simulink model "simulinkPark"  (R2024a)
settings: Solver=VariableStepAuto  StartTime=0.0  StopTime=11.5667  RelTol=1e-3
values from neighbouring files (symbols this model uses):
  posX = [sampleTimes',position(:,1)]    [main.m]
  posY = [sampleTimes',position(:,2)]    [main.m]
  posYaw = [sampleTimes',yaw]    [main.m]
libraries: sim3dautolib x11, visionsinks x2, sim3dcameralib x1, sim3dlib x1
settings Model: Creator=6000022946  LastModifiedBy=Administrator
settings RTWCC: GPUComputeCapability=3.5

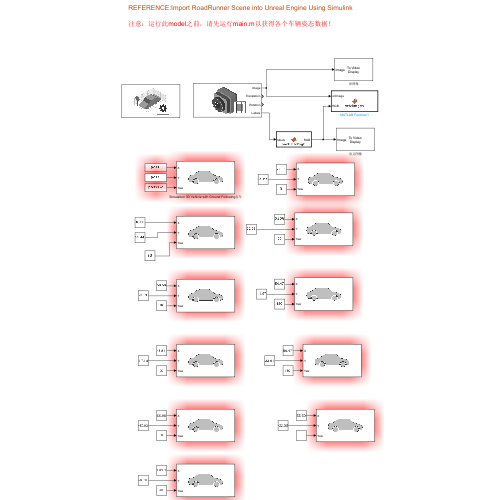
[thumbnail: Simulink's stored preview of the top-level diagram]
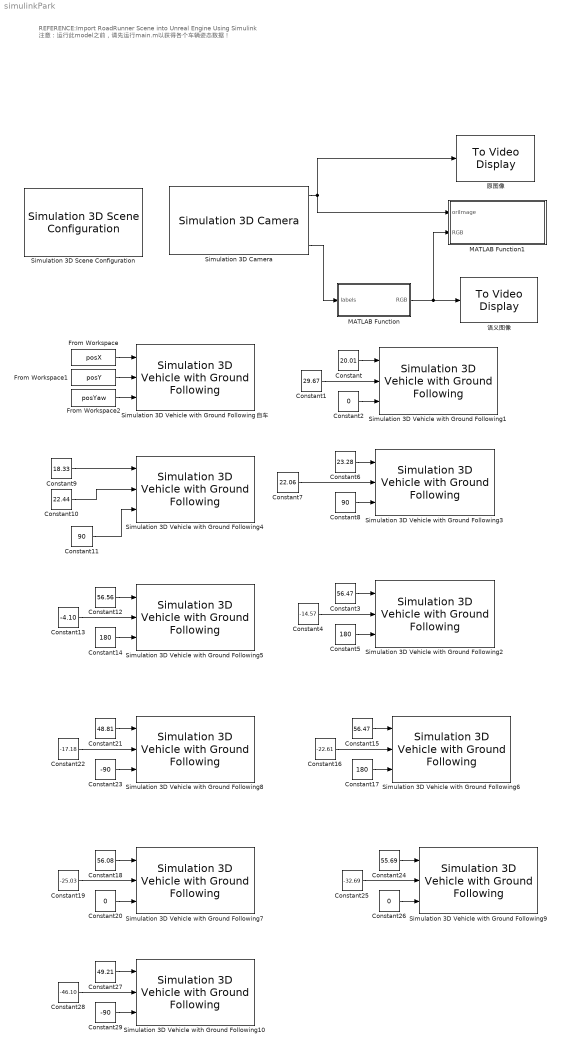
== system simulinkPark ==
  note: REFERENCE:Import RoadRunner Scene into Unreal Engine Using Simulink
      |
      | 注意：运行此model之前，请先运行main.m以获得各个车辆姿态数据！
  Constant : Constant  Value=20.01
  Constant1 : Constant  Value=29.67
  Constant10 : Constant  Value=22.44
  Constant11 : Constant  Value=90
  Constant12 : Constant  Value=56.56
  Constant13 : Constant  Value=-4.10
  Constant14 : Constant  Value=180
  Constant15 : Constant  Value=56.47
  Constant16 : Constant  Value=-22.61
  Constant17 : Constant  Value=180
  Constant18 : Constant  Value=56.08
  Constant19 : Constant  Value=-25.03
  Constant2 : Constant  Value=0
  Constant20 : Constant  Value=0
  Constant21 : Constant  Value=48.81
  Constant22 : Constant  Value=-17.18
  Constant23 : Constant  Value=-90
  Constant24 : Constant  Value=55.69
  Constant25 : Constant  Value=-32.69
  Constant26 : Constant  Value=0
  Constant27 : Constant  Value=49.21
  Constant28 : Constant  Value=-46.10
  Constant29 : Constant  Value=-90
  Constant3 : Constant  Value=56.47
  Constant4 : Constant  Value=-14.57
  Constant5 : Constant  Value=180
  Constant6 : Constant  Value=23.28
  Constant7 : Constant  Value=22.06
  Constant8 : Constant  Value=90
  Constant9 : Constant  Value=18.33
  From Workspace : FromWorkspace  VariableName=posX
  From Workspace1 : FromWorkspace  VariableName=posY
  From Workspace2 : FromWorkspace  VariableName=posYaw
  MATLAB Function : MATLAB Function  TreatAsAtomicUnit=on
  MATLAB Function1 : MATLAB Function  TreatAsAtomicUnit=on
  Simulation 3D Camera : sim3dcameralib/Simulation 3D Camera  Priority=1  sensorTag=Sim3dSensor5  sensorId=5  sensorName=Sim3dSensor5  vehTagList={'Scene Origin';'SimulinkVehicle10';'SimulinkVehicle11';'SimulinkVehicle12';'SimulinkVehicle13';'SimulinkVehicle4';'SimulinkVehicle5';'SimulinkVehicle6';'SimulinkVehicle7';'SimulinkVehicle8';'SimulinkVehicle9';'myEgoVehicle'}  vehTag=myEgoVehicle  mountLoc=Origin  offsetFlag=on  tmountOffset=[0, 0, 20]  extTmount=off  rmountOffset=[0, 90, 0]  extRmount=off  FocalLength=[1109, 1109]  OpticalCenter=[640, 360]  ImageSize=[720, 1280]  RadialDistortion=[0, 0]  TangentialDistortion=[0, 0]  SensorSkew=0  DepthOutportEnabled=off  SemanticOutportEnabled=on  TransformOutportEnabled=on  SampleTime=-1  mountPoint=[0 0 20]  mountOrientation=[0 -90 0]  aMode=3  ID=5
      settings: LibrarySourceBlock=drivingsim3d/Simulation 3D Camera
  Simulation 3D Scene Configuration : sim3dlib/Simulation 3D Scene Configuration  Priority=0  ProjectFormat=RoadRunner  SceneDesc=Straight road  ProjectName=C:\Program Files\MATLAB\R2024a\toolbox\shared\sim3d_projects\automotive_project_windows\UE\WindowsNoEditor\VehicleSimulation.exe  ScenePath=/Game/Maps/HwStrght  RoadRunnerProjectPath=./Exports/mySampleParking.fbx  EnableOpenDRIVE=off  vehTagList={'Custom';'Scene Origin';'SimulinkVehicle10';'SimulinkVehicle11';'SimulinkVehicle12';'SimulinkVehicle13';'SimulinkVehicle4';'SimulinkVehicle5';'SimulinkVehicle6';'SimulinkVehicle7';'SimulinkVehicle8';'SimulinkVehicle9';'myEgoVehicle'}  vehTag=Custom  FreeCameraInitialTranslation=[50, 0, 200]  FreeCameraDefaultInitialTranslation=[-6, 0, 2]  FreeCameraInitialRotation=[0, -90, 0]  FreeCameraDefaultInitialRotation=[0, -15, 0]  OpVisEn=off  Ts=1/60  EnableWindow=on  EnableRemoteAccess=off  EnableWeather=on  SunAzimuth=90  SunAltitude=40.0  EnableGeospatialSun=off  Latitude=0  Longitude=0  Date=2023-01-01  Time=10:30:00  GeoTimeZone=-5.0  SunDaylightSaving=off  wind=1  clouds=10  EnableVolumetricClouds=off  CloudCoverage=0  CloudAltitude=6  fog=57.0  rain=0.0  RaindropsEffect=off  SnowDensity=0  EnableGeospatial=off  UseTrueOrigin=off  OriginHeight=200  OriginLatitude=40.744652  OriginLongitude=-73.988864  MapStyle=Aerial  AdditionalAssetIDs=[]  UseAdvancedSunSky=off  SolarTime=11  TimeZone=-5  Day=21  Month=9  Year=2022  UseDaylightSavingTime=on  DSTStartDay=10  DSTStartMonth=3  DSTEndDay=3  DSTEndMonth=11  DSTSwitchHour=2  sensorTag=MainCamera1  sensorId=1  sensorName=MainCamera1  mountLoc=Origin  offsetFlag=off  tmountOffset=[0, 0, 0]  rmountOffset=[0, 0, 0]  HorizontalResolution=1280  VerticalResolution=720  HorizontalFOV=60  mountPoint=[0 0 0]  mountOrientation=[0 0 0]  aMode=3  ID=1  GeoTrigger=Inactive
      settings: LibrarySourceBlock=drivingsim3d/Simulation 3D Scene Configuration
  Simulation 3D Vehicle with Ground Following1 : sim3dautolib/Simulation 3D Vehicle with Ground Following  Priority=-1  PassVehMesh=Sport utility vehicle  MeshPath=/MathWorksAutomotiveContent/Vehicles/Muscle/Meshes/SK_MuscleCar.SK_MuscleCar  TrackWidth=1.9  WheelBase=3  WheelRadius=0.35  VehColor=Orange  InitialPos=[posX(1,2), posY(1,2), 0]  InitialRot=[0, 0, posYaw(1,2)]  ActorName=SimulinkVehicle4  SampleTime=-1  ActorType=SimulinkVehicle  ID=4  aMode=3  ActorTag=SimulinkVehicle4  CoordinateScheme=ISO  VehLightsControl=off  HeadlightColor=[ 1, 1, 1 ]  HighBeamIntensity=100000  LowBeamIntensity=60000  HighBeamConeAngle=70  LowBeamConeAngle=70  LeftHeadlightOrientation=[ 0, 0 ]  RightHeadlightOrientation=[ 0, 0 ]  BrakelightIntensity=500  ReverselightIntensity=500  SignallightIntensity=500  SignallightPeriod=1  SignalPulseWidth=50  TransformOutportEnabled=off
      settings: LibrarySourceBlock=drivingsim3d/Simulation 3D Vehicle with Ground Following
  Simulation 3D Vehicle with Ground Following10 : sim3dautolib/Simulation 3D Vehicle with Ground Following  Priority=-1  PassVehMesh=Muscle car  MeshPath=/MathWorksAutomotiveContent/Vehicles/Muscle/Meshes/SK_MuscleCar.SK_MuscleCar  TrackWidth=1.9  WheelBase=3  WheelRadius=0.35  VehColor=White  InitialPos=[posX(1,2), posY(1,2), 0]  InitialRot=[0, 0, posYaw(1,2)]  ActorName=SimulinkVehicle13  SampleTime=-1  ActorType=SimulinkVehicle  ID=13  aMode=3  ActorTag=SimulinkVehicle13  CoordinateScheme=ISO  VehLightsControl=off  HeadlightColor=[ 1, 1, 1 ]  HighBeamIntensity=100000  LowBeamIntensity=60000  HighBeamConeAngle=70  LowBeamConeAngle=70  LeftHeadlightOrientation=[ 0, 0 ]  RightHeadlightOrientation=[ 0, 0 ]  BrakelightIntensity=500  ReverselightIntensity=500  SignallightIntensity=500  SignallightPeriod=1  SignalPulseWidth=50  TransformOutportEnabled=off
      settings: LibrarySourceBlock=drivingsim3d/Simulation 3D Vehicle with Ground Following
  Simulation 3D Vehicle with Ground Following2 : sim3dautolib/Simulation 3D Vehicle with Ground Following  Priority=-1  PassVehMesh=Hatchback  MeshPath=/MathWorksAutomotiveContent/Vehicles/Muscle/Meshes/SK_MuscleCar.SK_MuscleCar  TrackWidth=1.9  WheelBase=3  WheelRadius=0.35  VehColor=Yellow  InitialPos=[posX(1,2), posY(1,2), 0]  InitialRot=[0, 0, posYaw(1,2)]  ActorName=SimulinkVehicle5  SampleTime=-1  ActorType=SimulinkVehicle  ID=5  aMode=3  ActorTag=SimulinkVehicle5  CoordinateScheme=ISO  VehLightsControl=off  HeadlightColor=[ 1, 1, 1 ]  HighBeamIntensity=100000  LowBeamIntensity=60000  HighBeamConeAngle=70  LowBeamConeAngle=70  LeftHeadlightOrientation=[ 0, 0 ]  RightHeadlightOrientation=[ 0, 0 ]  BrakelightIntensity=500  ReverselightIntensity=500  SignallightIntensity=500  SignallightPeriod=1  SignalPulseWidth=50  TransformOutportEnabled=off
      settings: LibrarySourceBlock=drivingsim3d/Simulation 3D Vehicle with Ground Following
  Simulation 3D Vehicle with Ground Following3 : sim3dautolib/Simulation 3D Vehicle with Ground Following  Priority=-1  PassVehMesh=Sedan  MeshPath=/MathWorksAutomotiveContent/Vehicles/Muscle/Meshes/SK_MuscleCar.SK_MuscleCar  TrackWidth=1.9  WheelBase=3  WheelRadius=0.35  VehColor=White  InitialPos=[posX(1,2), posY(1,2), 0]  InitialRot=[0, 0, posYaw(1,2)]  ActorName=SimulinkVehicle6  SampleTime=-1  ActorType=SimulinkVehicle  ID=6  aMode=3  ActorTag=SimulinkVehicle6  CoordinateScheme=ISO  VehLightsControl=off  HeadlightColor=[ 1, 1, 1 ]  HighBeamIntensity=100000  LowBeamIntensity=60000  HighBeamConeAngle=70  LowBeamConeAngle=70  LeftHeadlightOrientation=[ 0, 0 ]  RightHeadlightOrientation=[ 0, 0 ]  BrakelightIntensity=500  ReverselightIntensity=500  SignallightIntensity=500  SignallightPeriod=1  SignalPulseWidth=50  TransformOutportEnabled=off
      settings: LibrarySourceBlock=drivingsim3d/Simulation 3D Vehicle with Ground Following
  Simulation 3D Vehicle with Ground Following4 : sim3dautolib/Simulation 3D Vehicle with Ground Following  Priority=-1  PassVehMesh=Sedan  MeshPath=/MathWorksAutomotiveContent/Vehicles/Muscle/Meshes/SK_MuscleCar.SK_MuscleCar  TrackWidth=1.9  WheelBase=3  WheelRadius=0.35  VehColor=Blue  InitialPos=[posX(1,2), posY(1,2), 0]  InitialRot=[0, 0, posYaw(1,2)]  ActorName=SimulinkVehicle7  SampleTime=-1  ActorType=SimulinkVehicle  ID=7  aMode=3  ActorTag=SimulinkVehicle7  CoordinateScheme=ISO  VehLightsControl=off  HeadlightColor=[ 1, 1, 1 ]  HighBeamIntensity=100000  LowBeamIntensity=60000  HighBeamConeAngle=70  LowBeamConeAngle=70  LeftHeadlightOrientation=[ 0, 0 ]  RightHeadlightOrientation=[ 0, 0 ]  BrakelightIntensity=500  ReverselightIntensity=500  SignallightIntensity=500  SignallightPeriod=1  SignalPulseWidth=50  TransformOutportEnabled=off
      settings: LibrarySourceBlock=drivingsim3d/Simulation 3D Vehicle with Ground Following
  Simulation 3D Vehicle with Ground Following5 : sim3dautolib/Simulation 3D Vehicle with Ground Following  Priority=-1  PassVehMesh=Sedan  MeshPath=/MathWorksAutomotiveContent/Vehicles/Muscle/Meshes/SK_MuscleCar.SK_MuscleCar  TrackWidth=1.9  WheelBase=3  WheelRadius=0.35  VehColor=White  InitialPos=[posX(1,2), posY(1,2), 0]  InitialRot=[0, 0, posYaw(1,2)]  ActorName=SimulinkVehicle8  SampleTime=-1  ActorType=SimulinkVehicle  ID=8  aMode=3  ActorTag=SimulinkVehicle8  CoordinateScheme=ISO  VehLightsControl=off  HeadlightColor=[ 1, 1, 1 ]  HighBeamIntensity=100000  LowBeamIntensity=60000  HighBeamConeAngle=70  LowBeamConeAngle=70  LeftHeadlightOrientation=[ 0, 0 ]  RightHeadlightOrientation=[ 0, 0 ]  BrakelightIntensity=500  ReverselightIntensity=500  SignallightIntensity=500  SignallightPeriod=1  SignalPulseWidth=50  TransformOutportEnabled=off
      settings: LibrarySourceBlock=drivingsim3d/Simulation 3D Vehicle with Ground Following
  Simulation 3D Vehicle with Ground Following6 : sim3dautolib/Simulation 3D Vehicle with Ground Following  Priority=-1  PassVehMesh=Muscle car  MeshPath=/MathWorksAutomotiveContent/Vehicles/Muscle/Meshes/SK_MuscleCar.SK_MuscleCar  TrackWidth=1.9  WheelBase=3  WheelRadius=0.35  VehColor=White  InitialPos=[posX(1,2), posY(1,2), 0]  InitialRot=[0, 0, posYaw(1,2)]  ActorName=SimulinkVehicle9  SampleTime=-1  ActorType=SimulinkVehicle  ID=9  aMode=3  ActorTag=SimulinkVehicle9  CoordinateScheme=ISO  VehLightsControl=off  HeadlightColor=[ 1, 1, 1 ]  HighBeamIntensity=100000  LowBeamIntensity=60000  HighBeamConeAngle=70  LowBeamConeAngle=70  LeftHeadlightOrientation=[ 0, 0 ]  RightHeadlightOrientation=[ 0, 0 ]  BrakelightIntensity=500  ReverselightIntensity=500  SignallightIntensity=500  SignallightPeriod=1  SignalPulseWidth=50  TransformOutportEnabled=off
      settings: LibrarySourceBlock=drivingsim3d/Simulation 3D Vehicle with Ground Following
  Simulation 3D Vehicle with Ground Following7 : sim3dautolib/Simulation 3D Vehicle with Ground Following  Priority=-1  PassVehMesh=Small pickup truck  MeshPath=/MathWorksAutomotiveContent/Vehicles/Muscle/Meshes/SK_MuscleCar.SK_MuscleCar  TrackWidth=1.9  WheelBase=3  WheelRadius=0.35  VehColor=Black  InitialPos=[posX(1,2), posY(1,2), 0]  InitialRot=[0, 0, posYaw(1,2)]  ActorName=SimulinkVehicle10  SampleTime=-1  ActorType=SimulinkVehicle  ID=10  aMode=3  ActorTag=SimulinkVehicle10  CoordinateScheme=ISO  VehLightsControl=off  HeadlightColor=[ 1, 1, 1 ]  HighBeamIntensity=100000  LowBeamIntensity=60000  HighBeamConeAngle=70  LowBeamConeAngle=70  LeftHeadlightOrientation=[ 0, 0 ]  RightHeadlightOrientation=[ 0, 0 ]  BrakelightIntensity=500  ReverselightIntensity=500  SignallightIntensity=500  SignallightPeriod=1  SignalPulseWidth=50  TransformOutportEnabled=off
      settings: LibrarySourceBlock=drivingsim3d/Simulation 3D Vehicle with Ground Following
  Simulation 3D Vehicle with Ground Following8 : sim3dautolib/Simulation 3D Vehicle with Ground Following  Priority=-1  PassVehMesh=Box truck  MeshPath=/MathWorksAutomotiveContent/Vehicles/Muscle/Meshes/SK_MuscleCar.SK_MuscleCar  TrackWidth=1.9  WheelBase=3  WheelRadius=0.35  VehColor=Green  InitialPos=[posX(1,2), posY(1,2), 0]  InitialRot=[0, 0, posYaw(1,2)]  ActorName=SimulinkVehicle11  SampleTime=-1  ActorType=SimulinkVehicle  ID=11  aMode=3  ActorTag=SimulinkVehicle11  CoordinateScheme=ISO  VehLightsControl=off  HeadlightColor=[ 1, 1, 1 ]  HighBeamIntensity=100000  LowBeamIntensity=60000  HighBeamConeAngle=70  LowBeamConeAngle=70  LeftHeadlightOrientation=[ 0, 0 ]  RightHeadlightOrientation=[ 0, 0 ]  BrakelightIntensity=500  ReverselightIntensity=500  SignallightIntensity=500  SignallightPeriod=1  SignalPulseWidth=50  TransformOutportEnabled=off
      settings: LibrarySourceBlock=drivingsim3d/Simulation 3D Vehicle with Ground Following
  Simulation 3D Vehicle with Ground Following9 : sim3dautolib/Simulation 3D Vehicle with Ground Following  Priority=-1  PassVehMesh=Small pickup truck  MeshPath=/MathWorksAutomotiveContent/Vehicles/Muscle/Meshes/SK_MuscleCar.SK_MuscleCar  TrackWidth=1.9  WheelBase=3  WheelRadius=0.35  VehColor=White  InitialPos=[posX(1,2), posY(1,2), 0]  InitialRot=[0, 0, posYaw(1,2)]  ActorName=SimulinkVehicle12  SampleTime=-1  ActorType=SimulinkVehicle  ID=12  aMode=3  ActorTag=SimulinkVehicle12  CoordinateScheme=ISO  VehLightsControl=off  HeadlightColor=[ 1, 1, 1 ]  HighBeamIntensity=100000  LowBeamIntensity=60000  HighBeamConeAngle=70  LowBeamConeAngle=70  LeftHeadlightOrientation=[ 0, 0 ]  RightHeadlightOrientation=[ 0, 0 ]  BrakelightIntensity=500  ReverselightIntensity=500  SignallightIntensity=500  SignallightPeriod=1  SignalPulseWidth=50  TransformOutportEnabled=off
      settings: LibrarySourceBlock=drivingsim3d/Simulation 3D Vehicle with Ground Following
  Simulation 3D Vehicle with Ground Following自车 : sim3dautolib/Simulation 3D Vehicle with Ground Following  Priority=-1  PassVehMesh=Muscle car  MeshPath=/MathWorksAutomotiveContent/Vehicles/Muscle/Meshes/SK_MuscleCar.SK_MuscleCar  TrackWidth=1.9  WheelBase=3  WheelRadius=0.35  VehColor=Red  InitialPos=[posX(1,2), posY(1,2), 0]  InitialRot=[0, 0, posYaw(1,2)]  ActorName=myEgoVehicle  SampleTime=-1  ActorType=SimulinkVehicle  ID=C  aMode=3  ActorTag=myEgoVehicle  CoordinateScheme=ISO  VehLightsControl=off  HeadlightColor=[ 1, 1, 1 ]  HighBeamIntensity=100000  LowBeamIntensity=60000  HighBeamConeAngle=70  LowBeamConeAngle=70  LeftHeadlightOrientation=[ 0, 0 ]  RightHeadlightOrientation=[ 0, 0 ]  BrakelightIntensity=500  ReverselightIntensity=500  SignallightIntensity=500  SignallightPeriod=1  SignalPulseWidth=50  TransformOutportEnabled=off
      settings: LibrarySourceBlock=drivingsim3d/Simulation 3D Vehicle with Ground Following
  原图像 : visionsinks/To Video Display  windowSizeMode=Normal  openAtMdlStart=on  fullScreen=off  videoWindowX=50  videoWindowY=130  saveWindowSize=off  videoWindowWidth=1280  videoWindowHeight=720  inputColorFormat=RGB  inputType=Obsolete  imagePorts=One multidimensional signal  OutputDevice=On-screen video monitor  dataOrg=Column-major  isWindowOpen=off
  语义图像 : visionsinks/To Video Display  windowSizeMode=Normal  openAtMdlStart=on  fullScreen=off  videoWindowX=1257  videoWindowY=107  saveWindowSize=off  videoWindowWidth=1280  videoWindowHeight=720  inputColorFormat=RGB  inputType=Obsolete  imagePorts=One multidimensional signal  OutputDevice=On-screen video monitor  dataOrg=Column-major  isWindowOpen=off
  wires:
  Simulation 3D Camera/1 -> MATLAB Function1/1(oriImage), 原图像/1
  Simulation 3D Camera/4 -> MATLAB Function/1(labels)
  MATLAB Function/1(RGB) -> MATLAB Function1/2(RGB), 语义图像/1
  From Workspace/1 -> Simulation 3D Vehicle with Ground Following自车/1
  From Workspace2/1 -> Simulation 3D Vehicle with Ground Following自车/3
  From Workspace1/1 -> Simulation 3D Vehicle with Ground Following自车/2
  Constant/1 -> Simulation 3D Vehicle with Ground Following1/1
  Constant1/1 -> Simulation 3D Vehicle with Ground Following1/2
  Constant2/1 -> Simulation 3D Vehicle with Ground Following1/3
  Constant5/1 -> Simulation 3D Vehicle with Ground Following2/3
  Constant3/1 -> Simulation 3D Vehicle with Ground Following2/1
  Constant4/1 -> Simulation 3D Vehicle with Ground Following2/2
  Constant8/1 -> Simulation 3D Vehicle with Ground Following3/3
  Constant6/1 -> Simulation 3D Vehicle with Ground Following3/1
  Constant7/1 -> Simulation 3D Vehicle with Ground Following3/2
  Constant11/1 -> Simulation 3D Vehicle with Ground Following4/3
  Constant9/1 -> Simulation 3D Vehicle with Ground Following4/1
  Constant10/1 -> Simulation 3D Vehicle with Ground Following4/2
  Constant14/1 -> Simulation 3D Vehicle with Ground Following5/3
  Constant12/1 -> Simulation 3D Vehicle with Ground Following5/1
  Constant13/1 -> Simulation 3D Vehicle with Ground Following5/2
  Constant17/1 -> Simulation 3D Vehicle with Ground Following6/3
  Constant15/1 -> Simulation 3D Vehicle with Ground Following6/1
  Constant16/1 -> Simulation 3D Vehicle with Ground Following6/2
  Constant20/1 -> Simulation 3D Vehicle with Ground Following7/3
  Constant18/1 -> Simulation 3D Vehicle with Ground Following7/1
  Constant19/1 -> Simulation 3D Vehicle with Ground Following7/2
  Constant23/1 -> Simulation 3D Vehicle with Ground Following8/3
  Constant21/1 -> Simulation 3D Vehicle with Ground Following8/1
  Constant22/1 -> Simulation 3D Vehicle with Ground Following8/2
  Constant26/1 -> Simulation 3D Vehicle with Ground Following9/3
  Constant24/1 -> Simulation 3D Vehicle with Ground Following9/1
  Constant25/1 -> Simulation 3D Vehicle with Ground Following9/2
  Constant29/1 -> Simulation 3D Vehicle with Ground Following10/3
  Constant27/1 -> Simulation 3D Vehicle with Ground Following10/1
  Constant28/1 -> Simulation 3D Vehicle with Ground Following10/2

== matlab function simulinkPark/MATLAB Function ==
  data: labels input; RGB output
function RGB = sim3dlabel2rgb(labels)
% Convert semantic segmentation map captured during 3D simulation to RGB
% color image.

% Declare label2rgb function.
coder.extrinsic('label2rgb');

% Preallocate memory for RGB matrix.
RGB = coder.nullcopy(zeros(size(labels,1),size(labels,2),3,class(labels)));

% Define colormap using 3D simulation label IDs.
cmap = sim3dColormap;

% Convert labels to RGB color image.
RGB = label2rgb(labels, cmap,'c');

== matlab function simulinkPark/MATLAB Function1 ==
  data: oriImage input; RGB input
function writeImages(oriImage, RGB)
persistent inum
if isempty(inum)
    inum = 1;
end

% coder.extrinsic("imwrite");
% imwrite(oriImage,string(inum)+"_ori.jpg");
% imwrite(RGB,string(inum)+"_seg.jpg");
inum = inum+1;
end
